simulink model "planner_contral"  (R2023b)
settings: Solver=FixedStepAuto  StartTime=0  StopTime=inf  FixedStep=0.001  RelTol=1e-3
undefined symbols (not defined in the file): aubr, c_factor, cf, cr, iniObsHeading1, iniObsHeading2, iniObsPos1, iniObsPos2, KD_PID_distance, KD_PID_speed, KI_PID_distance, KI_PID_speed, KP_PID_distance, KP_PID_speed, la, lb, LQR_K1, LQR_K2, LQR_K3, LQR_K4, m, rack_displacement, refInfo_obs1, refInfo_obs2, right_wheel_ground, rightWaypoints, tablebr, vubr, vx_break_point
libraries: Solver_SF x1
(part 3 of 8)

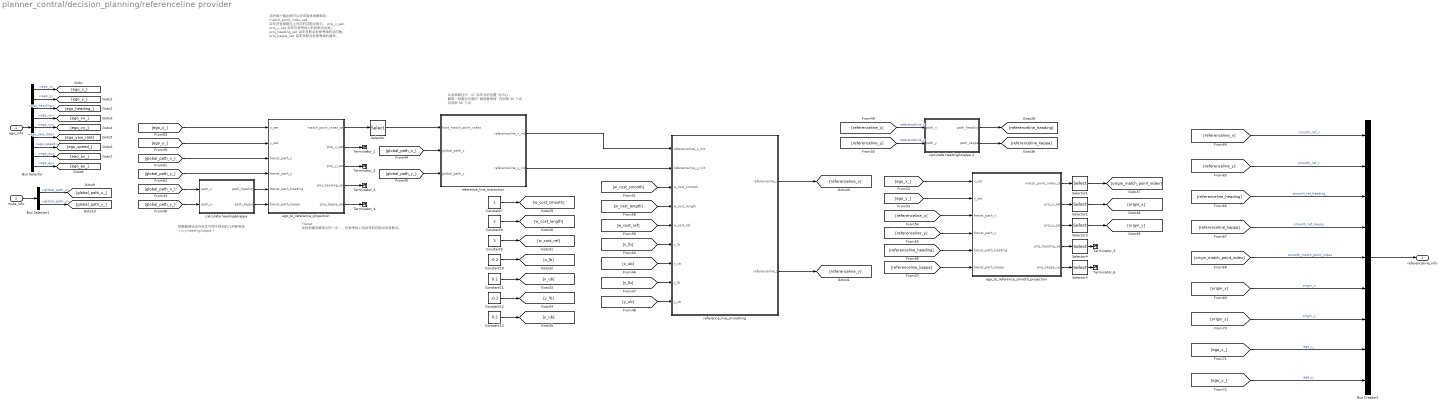
== system planner_contral/decision_planning/referenceline provider ==
  note: 从全局路径中，以“自车当前位置”为中心，
      | 截取一段固定长度的“局部参考线”
      | 向后取 30 个点
      | 向前取 90 个点
  note: 这时每个输出都可以非常具体地解释成：
      | match_point_index_set
      | 自车在全局路径上对应的匹配点索引。
      | proj_x_set, proj_y_set
      | 自车在参考线上的投影点坐标。
      | proj_heading_set
      | 自车投影点处参考线的切向角。
      | proj_kappa_set
      | 自车投影点处参考线的曲率。
  note: Frenet 坐标构建前最核心的一步：在参考线上找自车的匹配点和投影点。
  note: 把离散路径点升级生可用于规划的几何参考线
      | （x,y,heading,kappa）
  ego_info : Inport
  route_info : Inport  Port=2
  Bus Creator2 : BusCreator  Inputs=9
  Bus Selector : BusSelector  OutputSignals=ego_x,ego_y,ego_heading,ego_vx,ego_vy,ego_yaw_rate,ego_speed,ego_ax,ego_ay
  Bus Selector1 : BusSelector  OutputSignals=global_path_x,global_path_y
  Constant10 : Constant  Value=-0.2
  Constant11 : Constant  Value=0.2
  Constant12 : Constant  Value=-0.2
  Constant13 : Constant  Value=0.2
  Constant7 : Constant
  Constant8 : Constant  Value=2
  Constant9 : Constant  Value=3
  Selector{,1..5} (6 alike) : Selector  InputPortWidth=128  IndexOptions=Index vector (dialog)  Indices=1  OutputSizes=1
  Terminator_{1..6} (6 alike) : Terminator
  calculate heading&kappa : MATLAB Function  TreatAsAtomicUnit=on
  calculate heading&kappa 2 : MATLAB Function  TreatAsAtomicUnit=on
  ego_to_reference_projection : MATLAB Function  TreatAsAtomicUnit=on
  ego_to_reference_smooth_projection : MATLAB Function  TreatAsAtomicUnit=on
  reference_line_extraction : MATLAB Function  TreatAsAtomicUnit=on
  reference_line_smoothing : MATLAB Function  TreatAsAtomicUnit=on
  referenceline_info : Outport
  wires:
  ego_info/1 -> Bus Selector/1
  Bus Selector/7 -> [ego_speed_]  "<ego_speed>"
  Bus Selector/8 -> [eao_ax_]  "<ego_ax>"
  Bus Selector/9 -> [ego_ay_]  "<ego_ay>"
  Bus Selector/1 -> [ego_x_]  "<ego_x>"
  Bus Selector/2 -> [ego_y_]  "<ego_y>"
  Bus Selector/3 -> [ego_heading_]  "<ego_heading>"
  Bus Selector/4 -> [ego_vx_]  "<ego_vx>"
  Bus Selector/5 -> [ego_vy_]  "<ego_vy>"
  Bus Selector/6 -> [ego_yaw_rate]  "<ego_yaw_rate>"
  route_info/1 -> Bus Selector1/1
  Bus Selector1/1 -> [global_path_x_]  "<global_path_x>"
  Bus Selector1/2 -> [global_path_y_]  "<global_path_y>"
  Constant8/1 -> [w_cost_length]
  Constant11/1 -> [x_ub]
  [w_cost_ref] -> reference_line_smoothing/5(w_cost_ref)
  [y_lb] -> reference_line_smoothing/8(y_lb)
  [w_cost_smooth] -> reference_line_smoothing/3(w_cost_smooth)
  Constant9/1 -> [w_cost_ref]
  Constant10/1 -> [x_lb]
  reference_line_smoothing/2(referenceline_y) -> [referenceline_y]
  [global_path_y_] -> reference_line_extraction/3(global_path_y)
  [ego_x_] -> ego_to_reference_smooth_projection/1(x_set)
  calculate heading&kappa/1(path_heading) -> ego_to_reference_projection/5(frenet_path_heading)
  [ego_x_] -> ego_to_reference_projection/1(x_set)
  Constant7/1 -> [w_cost_smooth]
  Constant13/1 -> [y_ub]
  ego_to_reference_smooth_projection/5(proj_kappa_set) -> Selector5/1
  [referenceline_kappa] -> ego_to_reference_smooth_projection/6(frenet_path_kappa)
  ego_to_reference_projection/3(proj_y_set) -> Terminator_2/1
  [referenceline_y] -> ego_to_reference_smooth_projection/4(frenet_path_y)
  [referenceline_y] -> calculate heading&kappa 2/2(path_y)  "referenceline_y"
  [global_path_x_] -> ego_to_reference_projection/3(frenet_path_x)
  [global_path_y_] -> ego_to_reference_projection/4(frenet_path_y)
  [x_ub] -> reference_line_smoothing/7(x_ub)
  [global_path_x_] -> calculate heading&kappa/1(path_x)
  reference_line_extraction/2(referenceline_y_init) -> reference_line_smoothing/2(referenceline_y_init)
  ego_to_reference_projection/5(proj_kappa_set) -> Terminator_4/1
  ego_to_reference_projection/4(proj_heading_set) -> Terminator_3/1
  calculate heading&kappa 2/1(path_heading) -> [referenceline_heading]
  ego_to_reference_projection/2(proj_x_set) -> Terminator_1/1
  reference_line_smoothing/1(referenceline_x) -> [referenceline_x]
  Selector3/1 -> [origin_y]
  Selector2/1 -> [origin_x]
  ego_to_reference_smooth_projection/4(proj_heading_set) -> Selector4/1
  calculate heading&kappa 2/2(path_kappa) -> [referenceline_kappa]
  [referenceline_x] -> calculate heading&kappa 2/1(path_x)  "referenceline_x"
  [ego_y_] -> ego_to_reference_projection/2(y_set)
  [x_lb] -> reference_line_smoothing/6(x_lb)
  [referenceline_heading] -> ego_to_reference_smooth_projection/5(frenet_path_heading)
  ego_to_reference_smooth_projection/2(proj_x_set) -> Selector2/1
  calculate heading&kappa/2(path_kappa) -> ego_to_reference_projection/6(frenet_path_kappa)
  [y_ub] -> reference_line_smoothing/9(y_ub)
  [referenceline_x] -> ego_to_reference_smooth_projection/3(frenet_path_x)
  ego_to_reference_smooth_projection/1(match_point_index_set) -> Selector1/1
  [global_path_x_] -> reference_line_extraction/2(global_path_x)
  Selector5/1 -> Terminator_6/1
  reference_line_extraction/1(referenceline_x_init) -> reference_line_smoothing/1(referenceline_x_init)
  Selector4/1 -> Terminator_5/1
  [global_path_y_] -> calculate heading&kappa/2(path_y)
  ego_to_reference_smooth_projection/3(proj_y_set) -> Selector3/1
  ego_to_reference_projection/1(match_point_index_set) -> Selector/1
  Selector/1 -> reference_line_extraction/1(host_match_point_index)
  Constant12/1 -> [y_lb]
  [w_cost_length] -> reference_line_smoothing/4(w_cost_length)
  [ego_y_] -> ego_to_reference_smooth_projection/2(y_set)
  Selector1/1 -> [origin_match_point_index]
  [origin_match_point_index] -> Bus Creator2/5  "smooth_match_point_index"
  [ego_y_] -> Bus Creator2/9  "ego_y_"
  [ego_x_] -> Bus Creator2/8  "ego_x_"
  [referenceline_x] -> Bus Creator2/1  "smooth_ref_x"
  [referenceline_heading] -> Bus Creator2/3  "smooth_ref_heading_"
  [origin_x] -> Bus Creator2/6  "origin_x"
  [referenceline_kappa] -> Bus Creator2/4  "smooth_ref_kappa_"
  [origin_y] -> Bus Creator2/7  "origin_y"
  [referenceline_y] -> Bus Creator2/2  "smooth_ref_y"
  Bus Creator2/1 -> referenceline_info/1

== system planner_contral/control module/control main/chassic steering system ==
  LQR_final_angle : Inport
  Constant : Constant  Value=la
  Constant1 : Constant  Value=lb
  Constant17 : Constant  Value=c_factor
  Divide : Product  Inputs=*/
  Gain3 : Gain  Gain=180/pi
  Gain4 : Gain  Gain=360
  MATLAB Function : MATLAB Function  TreatAsAtomicUnit=on
  Saturation : Saturate  UpperLimit=70  LowerLimit=-70
  Saturation1 : Saturate  UpperLimit=1.2217  LowerLimit=-1.2217
  transfer right wheel angle to rack displancement : Lookup_n-D  NumberOfTableDimensions=1  BreakpointsForDimension1=right_wheel_ground  Table=rack_displacement  InternalRulePriority=Speed  RndMeth=Simplest
  lat_steer_sw[deg] : Outport
  wires:
  transfer right wheel angle to rack displancement/1 -> Divide/1
  Constant17/1 -> Divide/2
  Gain4/1 -> lat_steer_sw[deg]/1
  Divide/1 -> Gain4/1
  Saturation/1 -> transfer right wheel angle to rack displancement/1
  Constant/1 -> MATLAB Function/2(la)
  Gain3/1 -> Saturation/1
  Constant1/1 -> MATLAB Function/3(lb)
  LQR_final_angle/1 -> Saturation1/1
  Saturation1/1 -> MATLAB Function/1(u)
  MATLAB Function/1(right_steer) -> Gain3/1

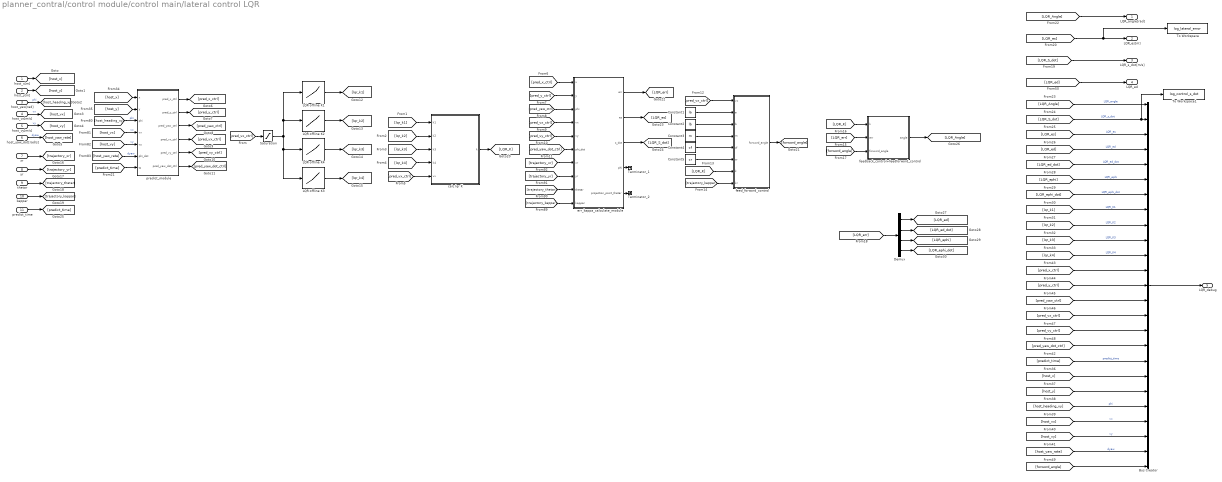
== system planner_contral/control module/control main/lateral control LQR ==
  host_x[m] : Inport
  host_y[m] : Inport  Port=2
  host_yaw[rad] : Inport  Port=3
  host_vx[m/s] : Inport  Port=4
  host_vy[m/s] : Inport  Port=5
  host_yaw_dot[rad/s] : Inport  Port=6
  xr : Inport  Port=7
  yr : Inport  Port=8
  thetar : Inport  Port=9
  kappar : Inport  Port=10
  predict_time : Inport  Port=11
  Bus Creator : BusCreator  Inputs=25
  Constant1 : Constant  Value=la
  Constant2 : Constant  Value=lb
  Constant3 : Constant  Value=m
  Constant4 : Constant  Value=cf
  Constant5 : Constant  Value=cr
  Demux : Demux
  LQR offline K1 : Lookup_n-D  NumberOfTableDimensions=1  BreakpointsForDimension1=vx_break_point  Table=LQR_K1  InternalRulePriority=Speed  RndMeth=Simplest
  LQR offline K2 : Lookup_n-D  NumberOfTableDimensions=1  BreakpointsForDimension1=vx_break_point  Table=LQR_K2  InternalRulePriority=Speed  RndMeth=Simplest
  LQR offline K3 : Lookup_n-D  NumberOfTableDimensions=1  BreakpointsForDimension1=vx_break_point  Table=LQR_K3  InternalRulePriority=Speed  RndMeth=Simplest
  LQR offline K4 : Lookup_n-D  NumberOfTableDimensions=1  BreakpointsForDimension1=vx_break_point  Table=LQR_K4  InternalRulePriority=Speed  RndMeth=Simplest
  Saturation : Saturate  UpperLimit=50  LowerLimit=0
  Terminator_1 : Terminator
  Terminator_2 : Terminator
  To Workspace : ToWorkspace  VariableName=log_lateral_error  SampleTime=-1
  To Workspace1 : ToWorkspace  VariableName=log_control_s_dot  SampleTime=-1
  calc lqr K : MATLAB Function  TreatAsAtomicUnit=on
  err_kappa_calculate_module : MATLAB Function  TreatAsAtomicUnit=on
  feed_forword_control : MATLAB Function  TreatAsAtomicUnit=on
  feedback_control+feedforword_control : MATLAB Function  TreatAsAtomicUnit=on
  predict_module : MATLAB Function  TreatAsAtomicUnit=on
  LQR_angle[rad] : Outport  VectorParamsAs1DForOutWhenUnconnected=off
  LQR_es[m] : Outport  Port=2  VectorParamsAs1DForOutWhenUnconnected=off
  LQR_s_dot[m/s] : Outport  Port=3  VectorParamsAs1DForOutWhenUnconnected=off
  LQR_ed : Outport  Port=4  VectorParamsAs1DForOutWhenUnconnected=off
  LQR_debug : Outport  Port=5  VectorParamsAs1DForOutWhenUnconnected=off
  wires:
  [host_vy] -> predict_module/5(vy)  "vy"
  [host_x] -> predict_module/1(x)
  [host_yaw_rate] -> predict_module/6(phi_dot)  "dyaw"
  [host_vx] -> predict_module/4(vx)  "vx"
  [host_y] -> predict_module/2(y)
  [host_heading_xy] -> predict_module/3(phi)  "phi"
  [predict_time] -> predict_module/7(ts)
  host_x[m]/1 -> [host_x]
  host_y[m]/1 -> [host_y]
  host_yaw[rad]/1 -> [host_heading_xy]  "phi"
  host_vx[m/s]/1 -> [host_vx]  "vx"
  host_vy[m/s]/1 -> [host_vy]  "vy"
  host_yaw_dot[rad/s]/1 -> [host_yaw_rate]  "dyaw"
  predict_module/1(pred_x_ctrl) -> [pred_x_ctrl]
  predict_module/2(pred_y_ctrl) -> [pred_y_ctrl]
  predict_module/3(pred_yaw_ctrl) -> [pred_yaw_ctrl]
  predict_module/4(pred_vx_ctrl) -> [pred_vx_ctrl]
  predict_module/5(pred_vy_ctrl) -> [pred_vy_ctrl]
  predict_module/6(pred_yaw_dot_ctrl) -> [pred_yaw_dot_ctrl]
  [pred_vx_ctrl] -> Saturation/1
  LQR offline K1/1 -> [lqr_k1]
  LQR offline K2/1 -> [lqr_k2]
  LQR offline K4/1 -> [lqr_k3]
  LQR offline K3/1 -> [lqr_k4]
  [pred_vx_ctrl] -> calc lqr K/5(vx)
  [lqr_k4] -> calc lqr K/4(k4)
  [lqr_k3] -> calc lqr K/3(k3)
  [lqr_k2] -> calc lqr K/2(k2)
  [lqr_k1] -> calc lqr K/1(k1)
  [pred_x_ctrl] -> err_kappa_calculate_module/1(x)
  [pred_y_ctrl] -> err_kappa_calculate_module/2(y)
  [pred_yaw_ctrl] -> err_kappa_calculate_module/3("phi ")
  [pred_vx_ctrl] -> err_kappa_calculate_module/4(vx)
  [pred_vy_ctrl] -> err_kappa_calculate_module/5(vy)
  [pred_yaw_dot_ctrl] -> err_kappa_calculate_module/6(phi_dot)
  xr/1 -> [trajectory_xr]
  yr/1 -> [trajectory_yr]
  thetar/1 -> [trajectory_thetar]
  kappar/1 -> [trajectory_kappar]
  [trajectory_xr] -> err_kappa_calculate_module/7(xr)
  [trajectory_yr] -> err_kappa_calculate_module/8(yr)
  [trajectory_kappar] -> err_kappa_calculate_module/10(kappar)
  [trajectory_thetar] -> err_kappa_calculate_module/9(thetar)
  [pred_vx_ctrl] -> feed_forword_control/1(vx)
  Constant1/1 -> feed_forword_control/2(a)
  Constant2/1 -> feed_forword_control/3(b)
  Constant3/1 -> feed_forword_control/4(m)
  Constant4/1 -> feed_forword_control/5(cf)
  Constant5/1 -> feed_forword_control/6(cr)
  calc lqr K/1(k) -> [LQR_K]
  [LQR_K] -> feed_forword_control/7(k)
  [trajectory_kappar] -> feed_forword_control/8(kr)
  feed_forword_control/1(forword_angle) -> [forword_angle]
  err_kappa_calculate_module/1(err) -> [LQR_err]
  [LQR_err] -> feedback_control+feedforword_control/2(err)
  [LQR_K] -> feedback_control+feedforword_control/1(k)
  [forword_angle] -> feedback_control+feedforword_control/3(forword_angle)
  [LQR_err] -> Demux/1
  err_kappa_calculate_module/2(es) -> [LQR_es]
  err_kappa_calculate_module/3(s_dot) -> [LQR_S_dot]
  [LQR_S_dot] -> LQR_s_dot[m/s]/1
  Saturation/1 -> LQR offline K3/1, LQR offline K4/1, LQR offline K2/1, LQR offline K1/1
  predict_time/1 -> [predict_time]
  Bus Creator/1 -> LQR_debug/1
  feedback_control+feedforword_control/1(angle) -> [LQR_Angle]
  [LQR_Angle] -> LQR_angle[rad]/1
  [LQR_Angle] -> Bus Creator/1  "LQR_angle"
  [LQR_S_dot] -> To Workspace1/1, Bus Creator/2  "LQR_s_dot"
  [LQR_es] -> Bus Creator/3  "LQR_es"
  Demux/1 -> [LQR_ed]
  Demux/2 -> [LQR_ed_dot]
  Demux/3 -> [LQR_ephi]
  Demux/4 -> [LQR_ephi_dot]
  [LQR_ed] -> Bus Creator/4  "LQR_ed"
  [LQR_ed_dot] -> Bus Creator/5  "LQR_ed_dot"
  [LQR_ephi] -> Bus Creator/6  "LQR_ephi"
  [LQR_ephi_dot] -> Bus Creator/7  "LQR_ephi_dot"
  [lqr_k1] -> Bus Creator/8  "LQR_K1"
  [lqr_k2] -> Bus Creator/9  "LQR_K2"
  [lqr_k3] -> Bus Creator/10  "LQR_K3"
  [lqr_k4] -> Bus Creator/11  "LQR_K4"
  [pred_x_ctrl] -> Bus Creator/12
  [pred_y_ctrl] -> Bus Creator/13
  [pred_yaw_ctrl] -> Bus Creator/14
  [pred_vx_ctrl] -> Bus Creator/15
  [pred_vy_ctrl] -> Bus Creator/16
  [pred_yaw_dot_ctrl] -> Bus Creator/17
  [predict_time] -> Bus Creator/18  "predict_time"
  [host_x] -> Bus Creator/19
  [host_y] -> Bus Creator/20
  [host_heading_xy] -> Bus Creator/21  "phi"
  [host_vx] -> Bus Creator/22  "vx"
  [host_vy] -> Bus Creator/23  "vy"
  [host_yaw_rate] -> Bus Creator/24  "dyaw"
  [forword_angle] -> Bus Creator/25
  [LQR_ed] -> LQR_ed/1
  err_kappa_calculate_module/4(phi) -> Terminator_1/1
  err_kappa_calculate_module/5(projection_point_thetar) -> Terminator_2/1
  [LQR_es] -> To Workspace/1, LQR_es[m]/1

== system planner_contral/control module/control main/longitudinal control double PID ==
  s_err[m] : Inport
  speed_desire[m/s] : Inport  Port=2
  accelerate desire[m/s^2] : Inport  Port=3
  host_speed[m/s] : Inport  Port=4
  host_s_dot[m/s] : Inport  Port=5
  KP_PID_distance : Inport  Port=6
  KI_PID_distance : Inport  Port=7
  KD_PID_distance : Inport  Port=8
  KP_PID_speed : Inport  Port=9
  KI_PID_speed : Inport  Port=10
  KD_PID_speed : Inport  Port=11
  2-D Lookup Table : Lookup_n-D  BreakpointsForDimension1=vubr  BreakpointsForDimension2=aubr  Table=tablebr  InternalRulePriority=Speed  RndMeth=Simplest
      settings: InputPortMap=u0,u1
  Add : Sum  Inputs=++-
  Add1 : Sum
  Bus Creator : BusCreator  Inputs=9
  Discrete Filter : DiscreteFilter
  MATLAB Function1 : MATLAB Function  TreatAsAtomicUnit=on
  Saturation : Saturate  UpperLimit=45  LowerLimit=-45
  Saturation1 : Saturate  UpperLimit=5  LowerLimit=-8
  To Workspace1 : ToWorkspace  VariableName=log_s_error  SampleTime=-1
  To Workspace3 : ToWorkspace  VariableName=log_host_s_dot  SaveFormat=Timeseries  SampleTime=-1
  To Workspace4 : ToWorkspace  VariableName=log_speed_desire  SampleTime=-1
  To Workspace5 : ToWorkspace  VariableName=log_accel_desire  SampleTime=-1
  discrete pid : Subsystem
  discrete pid1 : Subsystem
  throttle : Outport
  brake : Outport  Port=2
  longitudinal_debug : Outport  Port=3
  wires:
  2-D Lookup Table/1 -> MATLAB Function1/1(u)
  s_err[m]/1 -> To Workspace1/1, [s_err]
  speed_desire[m/s]/1 -> To Workspace4/1, [speed_desire]
  accelerate desire[m/s^2]/1 -> To Workspace5/1, [accelerate_desire]
  KP_PID_distance/1 -> [KP_PID_distance]
  KI_PID_distance/1 -> [KI_PID_distance]
  KD_PID_distance/1 -> [KD_PID_distance]
  KP_PID_speed/1 -> [KP_PID_speed]
  KI_PID_speed/1 -> [KI_PID_speed]
  KD_PID_speed/1 -> [KD_PID_speed]
  [s_err] -> Discrete Filter/1
  host_speed[m/s]/1 -> [host_speed]
  [speed_desire] -> Add/2
  Add/1 -> Saturation/1
  Saturation/1 -> discrete pid1/1(err)
  discrete pid1/1(pid_out) -> Add1/1
  [accelerate_desire] -> Add1/2
  Add1/1 -> Saturation1/1
  Saturation1/1 -> 2-D Lookup Table/2
  host_s_dot[m/s]/1 -> [host_s_dot]
  [host_s_dot] -> To Workspace3/1, Add/3
  [host_speed] -> 2-D Lookup Table/1
  MATLAB Function1/1(throttle) -> throttle/1
  MATLAB Function1/2(brake) -> brake/1
  [KP_PID_distance] -> Bus Creator/1  "KP_PID_distance"
  [KI_PID_distance] -> Bus Creator/2  "KI_PID_distance"
  [KD_PID_distance] -> Bus Creator/3  "KD_PID_distance"
  [KP_PID_speed] -> Bus Creator/4  "KP_PID_speed"
  [KI_PID_speed] -> Bus Creator/5  "KI_PID_speed"
  [KD_PID_speed] -> Bus Creator/6  "KD_PID_speed"
  [host_speed] -> Bus Creator/7  "host_speed"
  [s_err] -> Bus Creator/8  "s_err"
  [host_s_dot] -> Bus Creator/9  "host_s_dot"
  Bus Creator/1 -> longitudinal_debug/1
  Discrete Filter/1 -> discrete pid/1(err)
  [KP_PID_distance] -> discrete pid/2(kp)
  [KI_PID_distance] -> discrete pid/3(ki)
  [KD_PID_distance] -> discrete pid/4(kd)
  [KP_PID_speed] -> discrete pid1/2(kp)
  [KI_PID_speed] -> discrete pid1/3(ki)
  [KD_PID_speed] -> discrete pid1/4(kd)
  discrete pid/1(pid_out) -> Add/1

== system planner_contral/control module/control main/understeer compensate ==
  LQR_angle : Inport
  lateral err : Inport  Port=2
  Add : Sum  Inputs=+-
  Gain : Gain  Gain=0.01
  Manual Switch : ManualSwitch
  LQR_final_angle : Outport
  wires:
  lateral err/1 -> Gain/1
  Add/1 -> Manual Switch/2
  Manual Switch/1 -> LQR_final_angle/1
  LQR_angle/1 -> Add/1, Manual Switch/1
  Gain/1 -> Add/2

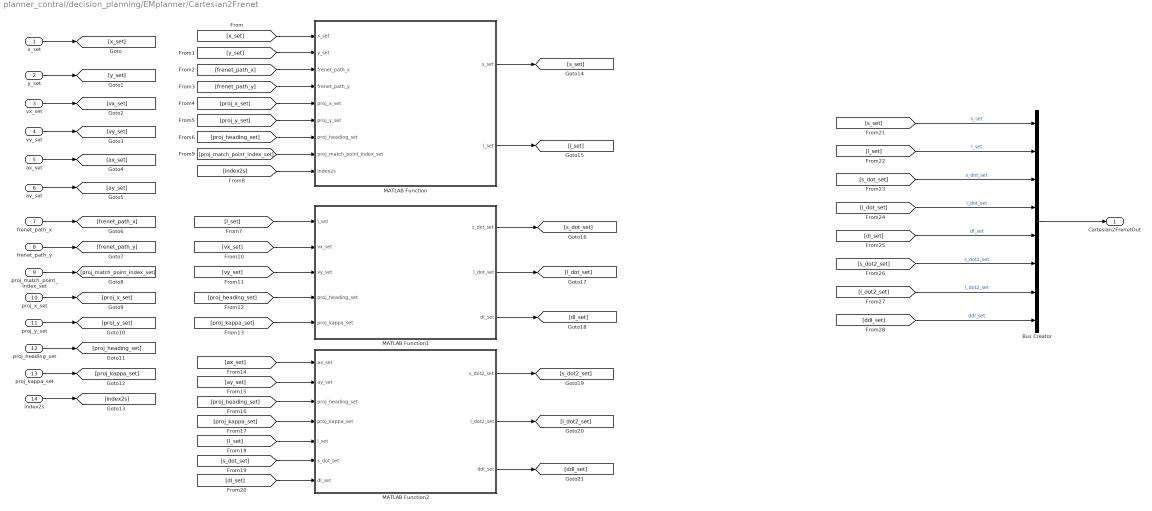
== system planner_contral/decision_planning/EMplanner/Cartesian2Frenet ==
  x_set : Inport
  y_set : Inport  Port=2
  vx_set : Inport  Port=3
  vy_set : Inport  Port=4
  ax_set : Inport  Port=5
  ay_set : Inport  Port=6
  frenet_path_x : Inport  Port=7
  frenet_path_y : Inport  Port=8
  proj_match_point_index_set : Inport  Port=9
  proj_x_set : Inport  Port=10
  proj_y_set : Inport  Port=11
  proj_heading_set : Inport  Port=12
  proj_kappa_set : Inport  Port=13
  index2s : Inport  Port=14
  Bus Creator : BusCreator  Inputs=8
  MATLAB Function : MATLAB Function  TreatAsAtomicUnit=on
  MATLAB Function1 : MATLAB Function  TreatAsAtomicUnit=on
  MATLAB Function2 : MATLAB Function  TreatAsAtomicUnit=on
  Cartesian2FrenetOut : Outport
  wires:
  x_set/1 -> [x_set]
  y_set/1 -> [y_set]
  vx_set/1 -> [vx_set]
  vy_set/1 -> [vy_set]
  ax_set/1 -> [ax_set]
  ay_set/1 -> [ay_set]
  frenet_path_x/1 -> [frenet_path_x]
  frenet_path_y/1 -> [frenet_path_y]
  proj_match_point_index_set/1 -> [proj_match_point_index_set]
  proj_x_set/1 -> [proj_x_set]
  proj_y_set/1 -> [proj_y_set]
  proj_heading_set/1 -> [proj_heading_set]
  proj_kappa_set/1 -> [proj_kappa_set]
  index2s/1 -> [index2s]
  [x_set] -> MATLAB Function/1(x_set)
  [y_set] -> MATLAB Function/2(y_set)
  [frenet_path_x] -> MATLAB Function/3(frenet_path_x)
  [frenet_path_y] -> MATLAB Function/4(frenet_path_y)
  [proj_x_set] -> MATLAB Function/5(proj_x_set)
  [proj_match_point_index_set] -> MATLAB Function/8(proj_match_point_index_set)
  [proj_y_set] -> MATLAB Function/6(proj_y_set)
  [proj_heading_set] -> MATLAB Function/7(proj_heading_set)
  [index2s] -> MATLAB Function/9(index2s)
  MATLAB Function/1(s_set) -> [s_set]
  MATLAB Function/2(l_set) -> [l_set]
  [l_set] -> MATLAB Function1/1(l_set)
  [vx_set] -> MATLAB Function1/2(vx_set)
  [vy_set] -> MATLAB Function1/3(vy_set)
  [proj_heading_set] -> MATLAB Function1/4(proj_heading_set)
  [proj_kappa_set] -> MATLAB Function1/5(proj_kappa_set)
  [ax_set] -> MATLAB Function2/1(ax_set)
  [ay_set] -> MATLAB Function2/2(ay_set)
  [proj_heading_set] -> MATLAB Function2/3(proj_heading_set)
  [proj_kappa_set] -> MATLAB Function2/4(proj_kappa_set)
  [l_set] -> MATLAB Function2/5(l_set)
  MATLAB Function1/1(s_dot_set) -> [s_dot_set]
  MATLAB Function1/2(l_dot_set) -> [l_dot_set]
  MATLAB Function1/3(dl_set) -> [dl_set]
  [s_dot_set] -> MATLAB Function2/6(s_dot_set)
  [dl_set] -> MATLAB Function2/7(dl_set)
  MATLAB Function2/1(s_dot2_set) -> [s_dot2_set]
  MATLAB Function2/2(l_dot2_set) -> [l_dot2_set]
  MATLAB Function2/3(ddl_set) -> [ddl_set]
  [s_set] -> Bus Creator/1  "s_set"
  [l_set] -> Bus Creator/2  "l_set"
  [s_dot_set] -> Bus Creator/3  "s_dot_set"
  [l_dot_set] -> Bus Creator/4  "l_dot_set"
  [dl_set] -> Bus Creator/5  "dl_set"
  [s_dot2_set] -> Bus Creator/6  "s_dot2_set"
  [l_dot2_set] -> Bus Creator/7  "l_dot2_set"
  [ddl_set] -> Bus Creator/8  "ddl_set"
  Bus Creator/1 -> Cartesian2FrenetOut/1

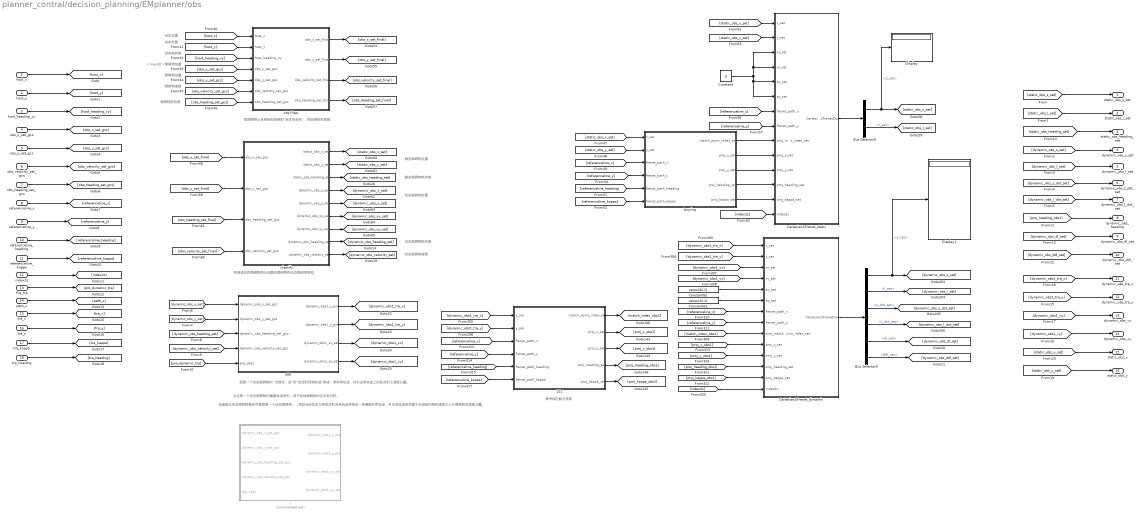
== system planner_contral/decision_planning/EMplanner/obs ==
  note: 参考线匹配与投影
  note: 该函数从动态障碍物集合中提取第一个动态障碍物，将其当前状态与预给定的未来轨迹拼接成一条离散时序轨迹，并为该轨迹附加基于当前航向角和速度大小计算得到的速度分量。
  note: 生成第一个动态障碍物的离散轨迹序列，用于后续障碍物时空关系分析。
  note: 把第一个动态障碍物的“当前状态”和“给定的预测轨迹”拼成一条时序轨迹，并为这条轨迹上的各点附上速度分量。
  note: 静态障碍物位置
  note: 把筛选后的障碍物再分成静态障碍物和动态障碍物两类。
  note: 把障碍物从全局坐标转换到“自车坐标系”，然后做矩形裁剪
  note: 自车位置
  note: 自车位置
  note: 自车航向角
  note: （max32）障碍物位置
  note: 障碍物位置
  note: 障碍物速度
  note: 障碍物航向角
  note: 静态障碍物航向角
  note: 动态障碍物位置
  note: 动态障碍物航向角
  note: 动态障碍物速度
  host_x : Inport
  host_y : Inport  Port=2
  host_heading_xy : Inport  Port=3
  obs_x_set_gcs : Inport  Port=4
  obs_y_set_gcs : Inport  Port=5
  obs_velocity_set_gcs : Inport  Port=6
  obs_heading_set_gcs : Inport  Port=7
  referenceline_x : Inport  Port=8
  referenceline_y : Inport  Port=9
  referenceline_heading : Inport  Port=10
  referenceline_kappa : Inport  Port=11
  index2s : Inport  Port=12
  Pre_tra : Inport  Port=13
  path_s : Inport  Port=14
  tra_x : Inport  Port=15
  tra_y : Inport  Port=16
  tra_kappa : Inport  Port=17
  tra_heaidng : Inport  Port=18
  000 : MATLAB Function  TreatAsAtomicUnit=on
  1 : MATLAB Function  Commented=on  TreatAsAtomicUnit=on
  111 : MATLAB Function  TreatAsAtomicUnit=on
  Bus Selector5 : BusSelector  OutputSignals=s_set,l_set
  Bus Selector9 : BusSelector  OutputSignals=s_set,l_set,s_dot_set,l_dot_set,dl_set,ddl_set
  Cartesian2Frenet_dynamic : Subsystem
  Cartesian2Frenet_static : Subsystem
  Constant : Constant  Value=0
  Constant62 : Constant  Value=zeros(32,1)
  Constant63 : Constant  Value=zeros(32,1)
  Display : Display
  Display1 : Display
  classify : MATLAB Function  TreatAsAtomicUnit=on
  obs filter : MATLAB Function  TreatAsAtomicUnit=on
  touying : MATLAB Function  TreatAsAtomicUnit=on
  static_obs_s_set : Outport
  static_obs_l_set : Outport  Port=2
  static_obs_heading_set : Outport  Port=3
  dynamic_obs_s_set : Outport  Port=4
  dynamic_obs_l_set : Outport  Port=5
  dynamic_obs_s_dot_set : Outport  Port=6
  dynamic_obs_l_dot_set : Outport  Port=7
  dynamic_obs_heading : Outport  Port=8
  dynamic_obs_dl_set : Outport  Port=9
  dynamic_obs_ddl_set : Outport  Port=10
  dynamic_obs_tra_x : Outport  Port=11
  dynamic_obs_tra_y : Outport  Port=12
  dynamic_obs_vx : Outport  Port=13
  dynamic_obs_vy : Outport  Port=14
  static_obs_x : Outport  Port=15
  static_obs_y : Outport  Port=16
  wires:
  Constant/1 -> Cartesian2Frenet_static/6(ay_set), Cartesian2Frenet_static/5(ax_set), Cartesian2Frenet_static/4(vy_set), Cartesian2Frenet_static/3(vx_set)
  [obs_x_set_gcs] -> obs filter/4(obs_x_set_gcs)
  [index2s] -> Cartesian2Frenet_static/14(index2s)
  [referenceline_y] -> Cartesian2Frenet_static/8(frenet_path_y)
  touying/5(proj_kappa_set) -> Cartesian2Frenet_static/13(proj_kappa_set)
  touying/4(proj_heading_set) -> Cartesian2Frenet_static/12(proj_heading_set)
  [referenceline_x] -> touying/3(frenet_path_x)
  obs filter/1(obs_x_set_final) -> [obs_x_set_final]
  obs filter/4(obs_heading_set_final) -> [obs_heading_set_final]
  [host_heading_xy] -> obs filter/3(host_heading_xy)
  classify/6(dynamic_obs_vx_set) -> [dynamic_obs_vx_set]
  [obs_y_set_final] -> classify/2(obs_y_set_gcs)
  classify/7(dynamic_obs_vy_set) -> [dynamic_obs_vy_set]
  [referenceline_y] -> touying/4(frenet_path_y)
  obs filter/3(obs_velocity_set_final) -> [obs_velocity_set_final]
  classify/1(static_obs_x_set) -> [static_obs_x_set]
  [obs_heading_set_gcs] -> obs filter/7(obs_heading_set_gcs)
  [referenceline_kappa] -> touying/6(frenet_path_kappa)
  [static_obs_x_set] -> Cartesian2Frenet_static/1(x_set)
  [static_obs_y_set] -> touying/2(y_set)
  [referenceline_x] -> Cartesian2Frenet_static/7(frenet_path_x)
  [obs_x_set_final] -> classify/1(obs_x_set_gcs)
  [obs_velocity_set_gcs] -> obs filter/6(obs_velocity_set_gcs)
  [host_y] -> obs filter/2(host_y)
  Bus Selector5/2 -> [static_obs_l_set]  "<l_set>"
  [referenceline_heading] -> touying/5(frenet_path_heading)
  obs filter/2(obs_y_set_final) -> [obs_y_set_final]
  Bus Selector5/1 -> Display/1, [static_obs_s_set]  "<s_set>"
  classify/4(dynamic_obs_x_set) -> [dynamic_obs_x_set]
  touying/2(proj_x_set) -> Cartesian2Frenet_static/10(proj_x_set)
  touying/3(proj_y_set) -> Cartesian2Frenet_static/11(proj_y_set)
  classify/5(dynamic_obs_y_set) -> [dynamic_obs_y_set]
  touying/1(match_point_index_set) -> Cartesian2Frenet_static/9(proj_match_point_index_set)
  [host_x] -> obs filter/1(host_x)
  [obs_y_set_gcs] -> obs filter/5(obs_y_set_gcs)
  Cartesian2Frenet_static/1(Cartesian2FrenetOut) -> Bus Selector5/1
  [static_obs_x_set] -> touying/1(x_set)
  classify/2(static_obs_y_set) -> [static_obs_y_set]
  [static_obs_y_set] -> Cartesian2Frenet_static/2(y_set)
  host_x/1 -> [host_x]
  host_y/1 -> [host_y]
  host_heading_xy/1 -> [host_heading_xy]
  obs_x_set_gcs/1 -> [obs_x_set_gcs]
  obs_y_set_gcs/1 -> [obs_y_set_gcs]
  obs_velocity_set_gcs/1 -> [obs_velocity_set_gcs]
  obs_heading_set_gcs/1 -> [obs_heading_set_gcs]
  referenceline_x/1 -> [referenceline_x]
  referenceline_y/1 -> [referenceline_y]
  referenceline_heading/1 -> [referenceline_heading]
  referenceline_kappa/1 -> [referenceline_kappa]
  index2s/1 -> [index2s]
  [static_obs_s_set] -> static_obs_s_set/1
  [static_obs_l_set] -> static_obs_l_set/1
  [dynamic_obs_l_dot_set] -> dynamic_obs_l_dot_set/1
  [dynamic_obs_s_dot_set] -> dynamic_obs_s_dot_set/1
  [dynamic_obs_l_set] -> dynamic_obs_l_set/1
  [dynamic_obs_s_set] -> dynamic_obs_s_set/1
  [obs_velocity_set_final] -> classify/4(obs_velocity_set_gcs)
  [obs_heading_set_final] -> classify/3(obs_heading_set_gcs)
  [index2s] -> Cartesian2Frenet_dynamic/14(index2s)
  000/2(dynamic_obs1_y_pre) -> [dynamic_obs1_tra_y]
  [referenceline_x] -> Cartesian2Frenet_dynamic/7(frenet_path_x)
  [referenceline_kappa] -> 111/6(frenet_path_kappa)
  [proj_y_obs1] -> Cartesian2Frenet_dynamic/11(proj_y_set)
  Bus Selector9/1 -> Display1/1, [dynamic_obs_s_set]  "<s_set>"
  Bus Selector9/3 -> [dynamic_obs_s_dot_set]  "<s_dot_set>"
  [dynamic_obs1_vy] -> Cartesian2Frenet_dynamic/4(vy_set)
  [dynamic_obs1_vx] -> Cartesian2Frenet_dynamic/3(vx_set)
  [proj_heading_obs1] -> Cartesian2Frenet_dynamic/12(proj_heading_set)
  [dynamic_obs1_tra_y] -> 111/2(y_set)
  [referenceline_y] -> 111/4(frenet_path_y)
  [proj_x_obs1] -> Cartesian2Frenet_dynamic/10(proj_x_set)
  Cartesian2Frenet_dynamic/1(Cartesian2FrenetOut) -> Bus Selector9/1
  Bus Selector9/4 -> [dynamic_obs_l_dot_set]  "<l_dot_set>"
  [match_index_obs1] -> Cartesian2Frenet_dynamic/9(proj_match_point_index_set)
  [dynamic_obs_x_set] -> 000/1(dynamic_obs_x_set_gcs)
  111/3(proj_y_set) -> [proj_y_obs1]
  Constant62/1 -> Cartesian2Frenet_dynamic/5(ax_set)
  000/1(dynamic_obs1_x_pre) -> [dynamic_obs1_tra_x]
  000/3(dynamic_obs1_vx_set) -> [dynamic_obs1_vx]
  111/1(match_point_index_set) -> [match_index_obs1]
  000/4(dynamic_obs1_vy_set) -> [dynamic_obs1_vy]
  Constant63/1 -> Cartesian2Frenet_dynamic/6(ay_set)
  [referenceline_y] -> Cartesian2Frenet_dynamic/8(frenet_path_y)
  [dynamic_obs1_tra_x] -> 111/1(x_set)
  111/5(proj_kappa_set) -> [proj_kappa_obs1]
  Bus Selector9/2 -> [dynamic_obs_l_set]  "<l_set>"
  [dynamic_obs1_tra_y] -> Cartesian2Frenet_dynamic/2(y_set)
  [referenceline_x] -> 111/3(frenet_path_x)
  [proj_kappa_obs1] -> Cartesian2Frenet_dynamic/13(proj_kappa_set)
  [referenceline_heading] -> 111/5(frenet_path_heading)
  111/2(proj_x_set) -> [proj_x_obs1]
  [dynamic_obs1_tra_x] -> Cartesian2Frenet_dynamic/1(x_set)
  111/4(proj_heading_set) -> [proj_heading_obs1]
  Pre_tra/1 -> [pro_dynamic_tra]
  path_s/1 -> [path_s]
  tra_y/1 -> [tra_y]
  tra_x/1 -> [tra_x]
  tra_heaidng/1 -> [tra_heading]
  tra_kappa/1 -> [tra_kappa]
  [dynamic_obs_y_set] -> 000/2(dynamic_obs_y_set_gcs)
  [dynamic_obs_heading_set] -> 000/3(dynamic_obs_heading_set_gcs)
  [dynamic_obs_velocity_set] -> 000/4(dynamic_obs_velocity_set_gcs)
  [pro_dynamic_tra] -> 000/5(pre_obs1)
  classify/8(dynamic_obs_heading_set) -> [dynamic_obs_heading_set]
  classify/9(dynamic_obs_velocity_set) -> [dynamic_obs_velocity_set]
  [proj_heading_obs1] -> dynamic_obs_heading/1
  Bus Selector9/5 -> [dynamic_obs_dl_set]  "<dl_set>"
  Bus Selector9/6 -> [dynamic_obs_ddl_set]  "<ddl_set>"
  [dynamic_obs_dl_set] -> dynamic_obs_dl_set/1
  [dynamic_obs_ddl_set] -> dynamic_obs_ddl_set/1
  classify/3(static_obs_heading_set) -> [static_obs_heading_set]
  [static_obs_heading_set] -> static_obs_heading_set/1
  [dynamic_obs1_vy] -> dynamic_obs_vy/1
  [dynamic_obs1_tra_y] -> dynamic_obs_tra_y/1
  [dynamic_obs1_vx] -> dynamic_obs_vx/1
  [dynamic_obs1_tra_x] -> dynamic_obs_tra_x/1
  [static_obs_x_set] -> static_obs_x/1
  [static_obs_y_set] -> static_obs_y/1

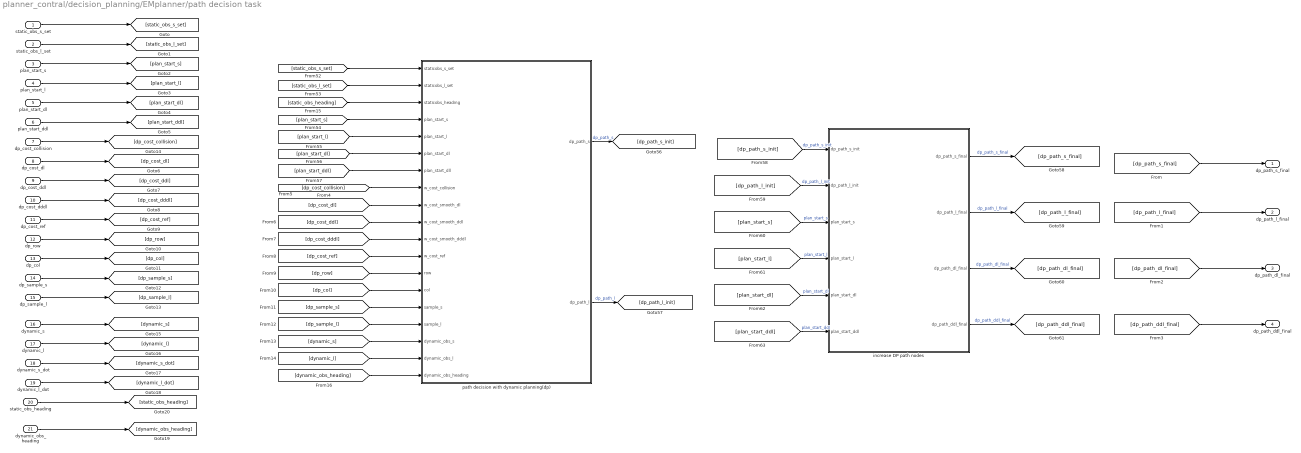
== system planner_contral/decision_planning/EMplanner/path decision task ==
  static_obs_s_set : Inport
  static_obs_l_set : Inport  Port=2
  plan_start_s : Inport  Port=3
  plan_start_l : Inport  Port=4
  plan_start_dl : Inport  Port=5
  plan_start_ddl : Inport  Port=6
  dp_cost_collision : Inport  Port=7
  dp_cost_dl : Inport  Port=8
  dp_cost_ddl : Inport  Port=9
  dp_cost_dddl : Inport  Port=10
  dp_cost_ref : Inport  Port=11
  dp_row : Inport  Port=12
  dp_col : Inport  Port=13
  dp_sample_s : Inport  Port=14
  dp_sample_l : Inport  Port=15
  dynamic_s : Inport  Port=16
  dynamic_l : Inport  Port=17
  dynamic_s_dot : Inport  Port=18
  dynamic_l_dot : Inport  Port=19
  static_obs_heading : Inport  Port=20
  dynamic_obs_heading : Inport  Port=21
  increase DP path nodes : MATLAB Function  TreatAsAtomicUnit=on
  path decision with dynamic planning(dp) : MATLAB Function  TreatAsAtomicUnit=on
  dp_path_s_final : Outport
  dp_path_l_final : Outport  Port=2
  dp_path_dl_final : Outport  Port=3
  dp_path_ddl_final : Outport  Port=4
  wires:
  [plan_start_s] -> path decision with dynamic planning(dp)/4(plan_start_s)
  path decision with dynamic planning(dp)/1(dp_path_s) -> [dp_path_s_init]  "dp_path_s"
  increase DP path nodes/2(dp_path_l_final) -> [dp_path_l_final]  "dp_path_l_final"
  [static_obs_l_set] -> path decision with dynamic planning(dp)/2(staticobs_l_set)
  [plan_start_ddl] -> path decision with dynamic planning(dp)/7(plan_start_dll)
  [plan_start_l] -> path decision with dynamic planning(dp)/5(plan_start_l)
  [static_obs_s_set] -> path decision with dynamic planning(dp)/1(staticobs_s_set)
  [plan_start_dl] -> increase DP path nodes/5(plan_start_dl)  "plan_start_dl"
  increase DP path nodes/4(dp_path_ddl_final) -> [dp_path_ddl_final]  "dp_path_ddl_final"
  increase DP path nodes/1(dp_path_s_final) -> [dp_path_s_final]  "dp_path_s_final"
  increase DP path nodes/3(dp_path_dl_final) -> [dp_path_dl_final]  "dp_path_dl_final"
  path decision with dynamic planning(dp)/2(dp_path_l) -> [dp_path_l_init]  "dp_path_l"
  [plan_start_l] -> increase DP path nodes/4(plan_start_l)  "plan_start_l"
  [plan_start_ddl] -> increase DP path nodes/6(plan_start_ddl)  "plan_start_ddl"
  [plan_start_dl] -> path decision with dynamic planning(dp)/6(plan_start_dl)
  [plan_start_s] -> increase DP path nodes/3(plan_start_s)  "plan_start_s"
  [dp_path_l_init] -> increase DP path nodes/2(dp_path_l_init)  "dp_path_l_init"
  [dp_path_s_init] -> increase DP path nodes/1(dp_path_s_init)  "dp_path_s_init"
  static_obs_s_set/1 -> [static_obs_s_set]
  static_obs_l_set/1 -> [static_obs_l_set]
  plan_start_s/1 -> [plan_start_s]
  plan_start_l/1 -> [plan_start_l]
  plan_start_dl/1 -> [plan_start_dl]
  plan_start_ddl/1 -> [plan_start_ddl]
  [dp_path_s_final] -> dp_path_s_final/1
  [dp_path_l_final] -> dp_path_l_final/1
  [dp_path_dl_final] -> dp_path_dl_final/1
  [dp_path_ddl_final] -> dp_path_ddl_final/1
  [dp_cost_collision] -> path decision with dynamic planning(dp)/8(w_cost_collision)
  [dp_cost_dl] -> path decision with dynamic planning(dp)/9(w_cost_smooth_dl)
  [dp_cost_ddl] -> path decision with dynamic planning(dp)/10(w_cost_smooth_ddl)
  [dp_cost_dddl] -> path decision with dynamic planning(dp)/11(w_cost_smooth_dddl)
  [dp_cost_ref] -> path decision with dynamic planning(dp)/12(w_cost_ref)
  [dp_row] -> path decision with dynamic planning(dp)/13(row)
  [dp_col] -> path decision with dynamic planning(dp)/14(col)
  [dp_sample_s] -> path decision with dynamic planning(dp)/15(sample_s)
  [dp_sample_l] -> path decision with dynamic planning(dp)/16(sample_l)
  dp_cost_dl/1 -> [dp_cost_dl]
  dp_cost_ddl/1 -> [dp_cost_ddl]
  dp_cost_dddl/1 -> [dp_cost_dddl]
  dp_cost_ref/1 -> [dp_cost_ref]
  dp_row/1 -> [dp_row]
  dp_col/1 -> [dp_col]
  dp_sample_l/1 -> [dp_sample_l]
  dp_sample_s/1 -> [dp_sample_s]
  dp_cost_collision/1 -> [dp_cost_collision]
  dynamic_l/1 -> [dynamic_l]
  dynamic_s/1 -> [dynamic_s]
  dynamic_l_dot/1 -> [dynamic_l_dot]
  dynamic_s_dot/1 -> [dynamic_s_dot]
  [dynamic_s] -> path decision with dynamic planning(dp)/17(dynamic_obs_s)
  [dynamic_l] -> path decision with dynamic planning(dp)/18(dynamic_obs_l)
  [static_obs_heading] -> path decision with dynamic planning(dp)/3(staticobs_heading)
  static_obs_heading/1 -> [static_obs_heading]
  dynamic_obs_heading/1 -> [dynamic_obs_heading]
  [dynamic_obs_heading] -> path decision with dynamic planning(dp)/19(dynamic_obs_heading)

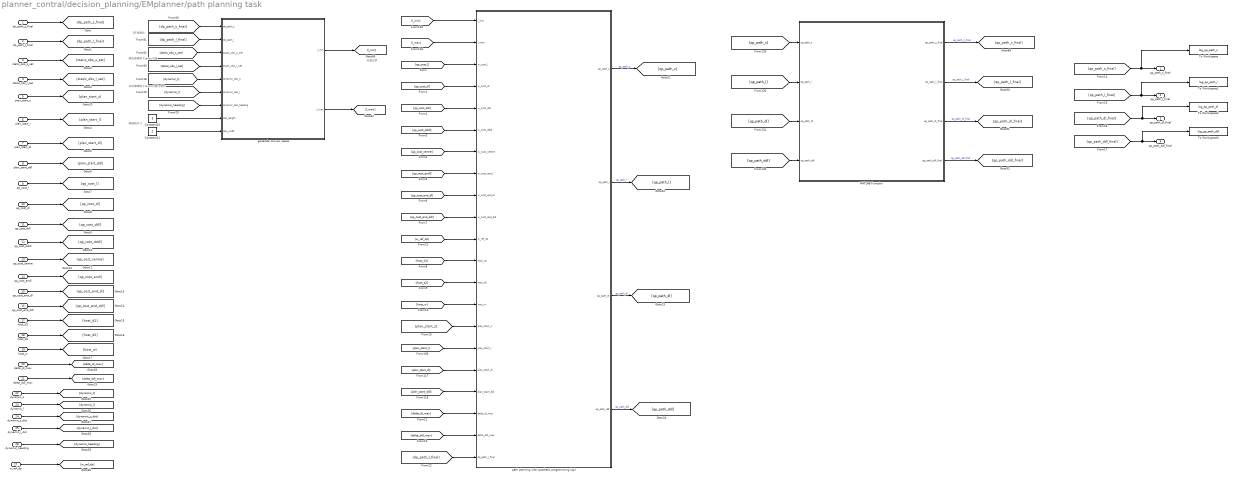
== system planner_contral/decision_planning/EMplanner/path planning task ==
  note: 走廊边界
  note: 障碍物尺寸
  note: 动态障碍物 Frenet 位置与朝向
  note: 静态障碍物 Frenet 位置
  note: DP粗路径
  dp_path_s_final : Inport
  dp_path_l_final : Inport  Port=2
  static_obs_s_set : Inport  Port=3
  static_obs_l_set : Inport  Port=4
  plan_start_s : Inport  Port=5
  plan_start_l : Inport  Port=6
  plan_start_dl : Inport  Port=7
  plan_start_ddl : Inport  Port=8
  qp_cost_l : Inport  Port=9
  qp_cost_dl : Inport  Port=10
  qp_cost_ddl : Inport  Port=11
  qp_cost_dddl : Inport  Port=12
  qp_cost_centre : Inport  Port=13
  qp_cost_endl : Inport  Port=14
  qp_cost_end_dl : Inport  Port=15
  qp_cost_end_ddl : Inport  Port=16
  host_d1 : Inport  Port=17
  host_d2 : Inport  Port=18
  host_w : Inport  Port=19
  delta_dl_max : Inport  Port=20
  delta_ddl_max : Inport  Port=21
  dynamic_s : Inport  Port=22
  dynamic_l : Inport  Port=23
  dynamic_s_dot : Inport  Port=24
  dynamic_l_dot : Inport  Port=25
  dynamic_heading : Inport  Port=26
  w_ref_dp : Inport  Port=27
  Constant10 : Constant  Value=5
  Constant11 : Constant  Value=2
  MATLAB Function : MATLAB Function  TreatAsAtomicUnit=on
  To Workspace : ToWorkspace  VariableName=log_qp_path_s  SampleTime=-1
  To Workspace1 : ToWorkspace  VariableName=log_qp_path_l  SampleTime=-1
  To Workspace2 : ToWorkspace  VariableName=log_qp_path_dl  SampleTime=-1
  To Workspace3 : ToWorkspace  VariableName=log_qp_path_ddl  SampleTime=-1
  generate convex space : MATLAB Function  TreatAsAtomicUnit=on
  path planning with quadratic programming (qp) : MATLAB Function  TreatAsAtomicUnit=on
  qp_path_s_final : Outport
  qp_path_l_final : Outport  Port=2
  qp_path_dl_final : Outport  Port=3
  qp_path_ddl_final : Outport  Port=4
  wires:
  generate convex space/2(l_max) -> [l_max]
  [static_obs_l_set] -> generate convex space/4(static_obs_l_set)
  [dp_path_s_final] -> generate convex space/1(dp_path_s)
  [plan_start_l] -> path planning with quadratic programming (qp)/16(plan_start_l)
  generate convex space/1(l_min) -> [l_min]
  [static_obs_s_set] -> generate convex space/3(static_obs_s_set)
  [dp_path_l_final] -> generate convex space/2(dp_path_l)
  [plan_start_dl] -> path planning with quadratic programming (qp)/17(plan_start_dl)
  [l_max] -> path planning with quadratic programming (qp)/2(l_max)
  [l_min] -> path planning with quadratic programming (qp)/1(l_min)
  [plan_start_ddl] -> path planning with quadratic programming (qp)/18(plan_start_ddl)
  dp_path_s_final/1 -> [dp_path_s_final]
  dp_path_l_final/1 -> [dp_path_l_final]
  static_obs_s_set/1 -> [static_obs_s_set]
  static_obs_l_set/1 -> [static_obs_l_set]
  plan_start_l/1 -> [plan_start_l]
  plan_start_dl/1 -> [plan_start_dl]
  plan_start_ddl/1 -> [plan_start_ddl]
  [qp_cost_l] -> path planning with quadratic programming (qp)/3(w_cost_l)
  [qp_cost_dl] -> path planning with quadratic programming (qp)/4(w_cost_dl)
  [qp_cost_ddl] -> path planning with quadratic programming (qp)/5(w_cost_ddl)
  [qp_cost_dddl] -> path planning with quadratic programming (qp)/6(w_cost_dddl)
  [qp_cost_centre] -> path planning with quadratic programming (qp)/7(w_cost_centre)
  [qp_cost_endl] -> path planning with quadratic programming (qp)/8(w_cost_end_l)
  [qp_cost_end_dl] -> path planning with quadratic programming (qp)/9(w_cost_end_dl)
  [qp_cost_end_ddl] -> path planning with quadratic programming (qp)/10(w_cost_end_ddl)
  [host_d1] -> path planning with quadratic programming (qp)/12(host_d1)
  [host_d2] -> path planning with quadratic programming (qp)/13(host_d2)
  [host_w] -> path planning with quadratic programming (qp)/14(host_w)
  qp_cost_l/1 -> [qp_cost_l]
  qp_cost_dl/1 -> [qp_cost_dl]
  qp_cost_ddl/1 -> [qp_cost_ddl]
  qp_cost_dddl/1 -> [qp_cost_dddl]
  qp_cost_centre/1 -> [qp_cost_centre]
  qp_cost_endl/1 -> [qp_cost_endl]
  qp_cost_end_dl/1 -> [qp_cost_end_dl]
  qp_cost_end_ddl/1 -> [qp_cost_end_ddl]
  host_d1/1 -> [host_d1]
  host_d2/1 -> [host_d2]
  host_w/1 -> [host_w]
  [delta_dl_max] -> path planning with quadratic programming (qp)/19(delta_dl_max)
  [delta_ddl_max] -> path planning with quadratic programming (qp)/20(delta_ddl_max)
  delta_dl_max/1 -> [delta_dl_max]
  delta_ddl_max/1 -> [delta_ddl_max]
  plan_start_s/1 -> [plan_start_s]
  [plan_start_s] -> path planning with quadratic programming (qp)/15(plan_start_s)
  MATLAB Function/1(qp_path_s_final) -> [qp_path_s_final]  "qp_path_s_final"
  MATLAB Function/3(qp_path_dl_final) -> [qp_path_dl_final]  "qp_path_dl_final"
  [qp_path_s] -> MATLAB Function/1(qp_path_s)
  [qp_path_ddl] -> MATLAB Function/4(qp_path_ddl)
  MATLAB Function/2(qp_path_l_final) -> [qp_path_l_final]  "qp_path_l_final"
  [qp_path_dl] -> MATLAB Function/3(qp_path_dl)
  MATLAB Function/4(qp_path_ddl_final) -> [qp_path_ddl_final]  "qp_path_ddl-final"
  [qp_path_l] -> MATLAB Function/2(qp_path_l)
  [qp_path_s_final] -> To Workspace/1, qp_path_s_final/1
  [qp_path_l_final] -> To Workspace1/1, qp_path_l_final/1
  [qp_path_dl_final] -> To Workspace2/1, qp_path_dl_final/1
  [qp_path_ddl_final] -> To Workspace3/1, qp_path_ddl_final/1
  path planning with quadratic programming (qp)/1(qp_path_s) -> [qp_path_s]  "qp_path_s"
  path planning with quadratic programming (qp)/2(qp_path_l) -> [qp_path_l]  "qp_path_l"
  path planning with quadratic programming (qp)/3(qp_path_dl) -> [qp_path_dl]  "qp_path_dl"
  path planning with quadratic programming (qp)/4(qp_path_ddl) -> [qp_path_ddl]  "qp_path_ddl"
  dynamic_l_dot/1 -> [dynamic_l_dot]
  dynamic_l/1 -> [dynamic_l]
  dynamic_s_dot/1 -> [dynamic_s_dot]
  dynamic_s/1 -> [dynamic_s]
  Constant11/1 -> generate convex space/9(obs_width)
  Constant10/1 -> generate convex space/8(obs_length)
  [dynamic_s] -> generate convex space/5(dynamic_obs_s)
  [dynamic_l] -> generate convex space/6(dynamic_obs_l)
  [dynamic_heading] -> generate convex space/7(dynamic_obs_heading)
  dynamic_heading/1 -> [dynamic_heading]
  w_ref_dp/1 -> [w_ref_dp]
  [w_ref_dp] -> path planning with quadratic programming (qp)/11(w_ref_dp)
  [dp_path_l_final] -> path planning with quadratic programming (qp)/21(dp_path_l_final)

== system planner_contral/control module/control main/longitudinal control double PID/discrete pid ==
  err : Inport
  kp : Inport  Port=2
  ki : Inport  Port=3
  kd : Inport  Port=4
  Add2 : Sum  Inputs=+++
  Add3 : Sum
  Add4 : Sum  Inputs=+-
  Delay3 : Delay  DelayLength=1
  Delay4 : Delay  DelayLength=1
  Divide : Product  Inputs=**
  Divide1 : Product  Inputs=**
  Divide2 : Product  Inputs=**
  Gain : Gain  Gain=0.01
  pid_out : Outport
  wires:
  [KD_PID_distance] -> Divide2/2
  err/1 -> Delay4/1, Divide/2, Add3/1, Add4/1
  Divide/1 -> Add2/1
  Divide2/1 -> Add2/3
  Add3/1 -> Gain/1, Divide1/1
  Delay4/1 -> Add4/2
  [KP_PID_distance] -> Divide/1
  Divide1/1 -> Add2/2
  Delay3/1 -> Add3/2
  [KI_PID_distance] -> Divide1/2
  Add4/1 -> Divide2/1
  Add2/1 -> pid_out/1
  kp/1 -> [KP_PID_distance]
  ki/1 -> [KI_PID_distance]
  kd/1 -> [KD_PID_distance]
  Gain/1 -> Delay3/1

== system planner_contral/control module/control main/longitudinal control double PID/discrete pid1 ==
  err : Inport
  kp : Inport  Port=2
  ki : Inport  Port=3
  kd : Inport  Port=4
  Add2 : Sum  Inputs=+++
  Add3 : Sum
  Add4 : Sum  Inputs=+-
  Delay3 : Delay  DelayLength=1
  Delay4 : Delay  DelayLength=1
  Divide : Product  Inputs=**
  Divide1 : Product  Inputs=**
  Divide2 : Product  Inputs=**
  Gain : Gain  Gain=0.01
  pid_out : Outport
  wires:
  Gain/1 -> Delay3/1
  kd/1 -> [KD_PID_distance]
  ki/1 -> [KI_PID_distance]
  kp/1 -> [KP_PID_distance]
  Add2/1 -> pid_out/1
  Add4/1 -> Divide2/1
  [KI_PID_distance] -> Divide1/2
  Delay3/1 -> Add3/2
  Divide1/1 -> Add2/2
  [KP_PID_distance] -> Divide/1
  Delay4/1 -> Add4/2
  Add3/1 -> Divide1/1, Gain/1
  Divide2/1 -> Add2/3
  Divide/1 -> Add2/1
  err/1 -> Add4/1, Add3/1, Divide/2, Delay4/1
  [KD_PID_distance] -> Divide2/2

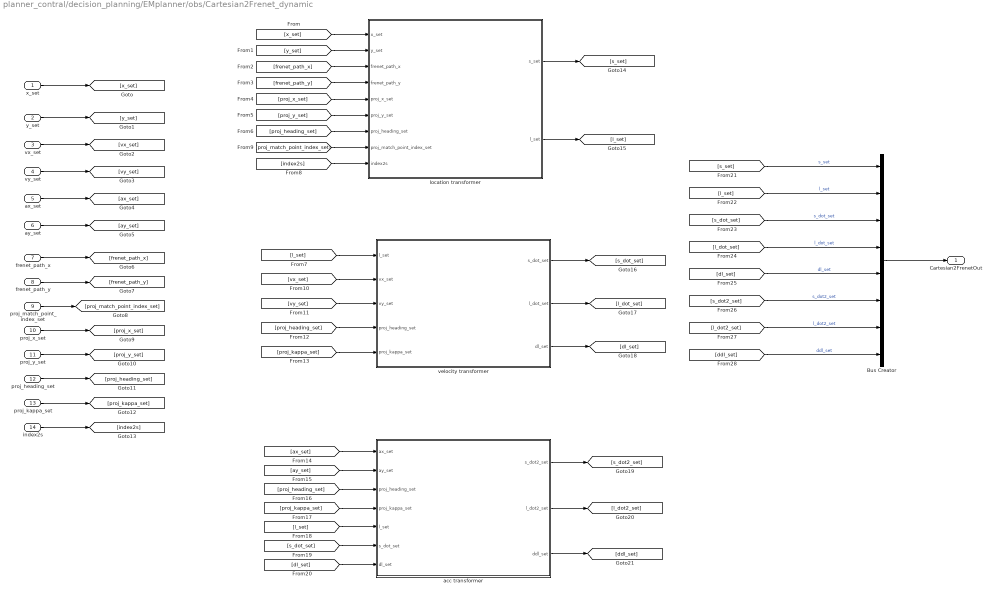
== system planner_contral/decision_planning/EMplanner/obs/Cartesian2Frenet_dynamic ==
  x_set : Inport
  y_set : Inport  Port=2
  vx_set : Inport  Port=3
  vy_set : Inport  Port=4
  ax_set : Inport  Port=5
  ay_set : Inport  Port=6
  frenet_path_x : Inport  Port=7
  frenet_path_y : Inport  Port=8
  proj_match_point_index_set : Inport  Port=9
  proj_x_set : Inport  Port=10
  proj_y_set : Inport  Port=11
  proj_heading_set : Inport  Port=12
  proj_kappa_set : Inport  Port=13
  index2s : Inport  Port=14
  Bus Creator : BusCreator  Inputs=8
  acc transformer : MATLAB Function  TreatAsAtomicUnit=on
  location transformer : MATLAB Function  TreatAsAtomicUnit=on
  velocity transformer : MATLAB Function  TreatAsAtomicUnit=on
  Cartesian2FrenetOut : Outport
  wires:
  Bus Creator/1 -> Cartesian2FrenetOut/1
  [ddl_set] -> Bus Creator/8  "ddl_set"
  [l_dot2_set] -> Bus Creator/7  "l_dot2_set"
  [s_dot2_set] -> Bus Creator/6  "s_dot2_set"
  [dl_set] -> Bus Creator/5  "dl_set"
  [l_dot_set] -> Bus Creator/4  "l_dot_set"
  [s_dot_set] -> Bus Creator/3  "s_dot_set"
  [l_set] -> Bus Creator/2  "l_set"
  [s_set] -> Bus Creator/1  "s_set"
  acc transformer/3(ddl_set) -> [ddl_set]
  acc transformer/2(l_dot2_set) -> [l_dot2_set]
  acc transformer/1(s_dot2_set) -> [s_dot2_set]
  [dl_set] -> acc transformer/7(dl_set)
  [s_dot_set] -> acc transformer/6(s_dot_set)
  velocity transformer/3(dl_set) -> [dl_set]
  velocity transformer/2(l_dot_set) -> [l_dot_set]
  velocity transformer/1(s_dot_set) -> [s_dot_set]
  [l_set] -> acc transformer/5(l_set)
  [proj_kappa_set] -> acc transformer/4(proj_kappa_set)
  [proj_heading_set] -> acc transformer/3(proj_heading_set)
  [ay_set] -> acc transformer/2(ay_set)
  [ax_set] -> acc transformer/1(ax_set)
  [proj_kappa_set] -> velocity transformer/5(proj_kappa_set)
  [proj_heading_set] -> velocity transformer/4(proj_heading_set)
  [vy_set] -> velocity transformer/3(vy_set)
  [vx_set] -> velocity transformer/2(vx_set)
  [l_set] -> velocity transformer/1(l_set)
  location transformer/2(l_set) -> [l_set]
  location transformer/1(s_set) -> [s_set]
  [index2s] -> location transformer/9(index2s)
  [proj_heading_set] -> location transformer/7(proj_heading_set)
  [proj_y_set] -> location transformer/6(proj_y_set)
  [proj_match_point_index_set] -> location transformer/8(proj_match_point_index_set)
  [proj_x_set] -> location transformer/5(proj_x_set)
  [frenet_path_y] -> location transformer/4(frenet_path_y)
  [frenet_path_x] -> location transformer/3(frenet_path_x)
  [y_set] -> location transformer/2(y_set)
  [x_set] -> location transformer/1(x_set)
  index2s/1 -> [index2s]
  proj_kappa_set/1 -> [proj_kappa_set]
  proj_heading_set/1 -> [proj_heading_set]
  proj_y_set/1 -> [proj_y_set]
  proj_x_set/1 -> [proj_x_set]
  proj_match_point_index_set/1 -> [proj_match_point_index_set]
  frenet_path_y/1 -> [frenet_path_y]
  frenet_path_x/1 -> [frenet_path_x]
  ay_set/1 -> [ay_set]
  ax_set/1 -> [ax_set]
  vy_set/1 -> [vy_set]
  vx_set/1 -> [vx_set]
  y_set/1 -> [y_set]
  x_set/1 -> [x_set]

== system planner_contral/decision_planning/EMplanner/obs/Cartesian2Frenet_static ==
  x_set : Inport
  y_set : Inport  Port=2
  vx_set : Inport  Port=3
  vy_set : Inport  Port=4
  ax_set : Inport  Port=5
  ay_set : Inport  Port=6
  frenet_path_x : Inport  Port=7
  frenet_path_y : Inport  Port=8
  proj_match_point_index_set : Inport  Port=9
  proj_x_set : Inport  Port=10
  proj_y_set : Inport  Port=11
  proj_heading_set : Inport  Port=12
  proj_kappa_set : Inport  Port=13
  index2s : Inport  Port=14
  Bus Creator : BusCreator  Inputs=8
  From10 : From  Commented=on  GotoTag=vx_set
  From11 : From  Commented=on  GotoTag=vy_set
  From12 : From  Commented=on  GotoTag=proj_heading_set
  From13 : From  Commented=on  GotoTag=proj_kappa_set
  From14 : From  Commented=on  GotoTag=ax_set
  From15 : From  Commented=on  GotoTag=ay_set
  From16 : From  Commented=on  GotoTag=proj_heading_set
  From17 : From  Commented=on  GotoTag=proj_kappa_set
  From18 : From  Commented=on  GotoTag=l_set
  From19 : From  Commented=on  GotoTag=s_dot_set
  From20 : From  Commented=on  GotoTag=dl_set
  From7 : From  Commented=on  GotoTag=l_set
  MATLAB Function : MATLAB Function  TreatAsAtomicUnit=on
  MATLAB Function1 : MATLAB Function  Commented=on  TreatAsAtomicUnit=on
  MATLAB Function2 : MATLAB Function  Commented=on  TreatAsAtomicUnit=on
  Cartesian2FrenetOut : Outport
  wires:
  Bus Creator/1 -> Cartesian2FrenetOut/1
  [ddl_set] -> Bus Creator/8  "ddl_set"
  [l_dot2_set] -> Bus Creator/7  "l_dot2_set"
  [s_dot2_set] -> Bus Creator/6  "s_dot2_set"
  [dl_set] -> Bus Creator/5  "dl_set"
  [l_dot_set] -> Bus Creator/4  "l_dot_set"
  [s_dot_set] -> Bus Creator/3  "s_dot_set"
  [l_set] -> Bus Creator/2  "l_set"
  [s_set] -> Bus Creator/1  "s_set"
  MATLAB Function2/3(ddl_set) -> [ddl_set]
  MATLAB Function2/2(l_dot2_set) -> [l_dot2_set]
  MATLAB Function2/1(s_dot2_set) -> [s_dot2_set]
  From20/1 -> MATLAB Function2/7(dl_set)
  From19/1 -> MATLAB Function2/6(s_dot_set)
  MATLAB Function1/3(dl_set) -> [dl_set]
  MATLAB Function1/2(l_dot_set) -> [l_dot_set]
  MATLAB Function1/1(s_dot_set) -> [s_dot_set]
  From18/1 -> MATLAB Function2/5(l_set)
  From17/1 -> MATLAB Function2/4(proj_kappa_set)
  From16/1 -> MATLAB Function2/3(proj_heading_set)
  From15/1 -> MATLAB Function2/2(ay_set)
  From14/1 -> MATLAB Function2/1(ax_set)
  From13/1 -> MATLAB Function1/5(proj_kappa_set)
  From12/1 -> MATLAB Function1/4(proj_heading_set)
  From11/1 -> MATLAB Function1/3(vy_set)
  From10/1 -> MATLAB Function1/2(vx_set)
  From7/1 -> MATLAB Function1/1(l_set)
  MATLAB Function/2(l_set) -> [l_set]
  MATLAB Function/1(s_set) -> [s_set]
  [index2s] -> MATLAB Function/9(index2s)
  [proj_heading_set] -> MATLAB Function/7(proj_heading_set)
  [proj_y_set] -> MATLAB Function/6(proj_y_set)
  [proj_match_point_index_set] -> MATLAB Function/8(proj_match_point_index_set)
  [proj_x_set] -> MATLAB Function/5(proj_x_set)
  [frenet_path_y] -> MATLAB Function/4(frenet_path_y)
  [frenet_path_x] -> MATLAB Function/3(frenet_path_x)
  [y_set] -> MATLAB Function/2(y_set)
  [x_set] -> MATLAB Function/1(x_set)
  index2s/1 -> [index2s]
  proj_kappa_set/1 -> [proj_kappa_set]
  proj_heading_set/1 -> [proj_heading_set]
  proj_y_set/1 -> [proj_y_set]
  proj_x_set/1 -> [proj_x_set]
  proj_match_point_index_set/1 -> [proj_match_point_index_set]
  frenet_path_y/1 -> [frenet_path_y]
  frenet_path_x/1 -> [frenet_path_x]
  ay_set/1 -> [ay_set]
  ax_set/1 -> [ax_set]
  vy_set/1 -> [vy_set]
  vx_set/1 -> [vx_set]
  y_set/1 -> [y_set]
  x_set/1 -> [x_set]

== matlab function planner_contral/decision_planning/EMplanner/path planning task/MATLAB Function ==
  data: qp_path_s input; qp_path_s_final output; qp_path_l input; qp_path_dl input; qp_path_ddl input; qp_path_l_final output; qp_path_dl_final output; qp_path_ddl_final output
function [qp_path_s_final,qp_path_l_final, qp_path_dl_final,qp_path_ddl_final] = fcn(qp_path_s,qp_path_l,qp_path_dl,qp_path_ddl)
% 该函数将增密qp_path
n_init = 20;
% 增密的点的个数
n = 501;
% 输出初始化
qp_path_s_final = zeros(n,1);
qp_path_l_final = zeros(n,1);
qp_path_dl_final = zeros(n,1);
qp_path_ddl_final = zeros(n,1);
ds = (qp_path_s(end) - qp_path_s(1))/(n-1);
index = 1;
for i = 1:n
    x = qp_path_s(1) + (i-1) * ds;
    qp_path_s_final(i) = x;
    while x >= qp_path_s(index)
        index = index + 1;
        if index == n_init
            break;
        end
    end
    % while 循环退出的条件是x<qp_path_s(index)，所以x对应的前一个s的编号是index-1 后一个编号是index
    pre = index - 1;
    cur = index;
    % 计算前一个点的l l' l'' ds 和后一个点的 l''
    delta_s = x - qp_path_s(pre);
    l_pre = qp_path_l(pre);
    dl_pre = qp_path_dl(pre);
    ddl_pre = qp_path_ddl(pre);
    ddl_cur = qp_path_ddl(cur);
    % 分段加加速度优化 
    qp_path_l_final(i) = l_pre + dl_pre * delta_s + (1/3)* ddl_pre * delta_s^2 + (1/6) * ddl_cur * delta_s^2;
    qp_path_dl_final(i) = dl_pre + 0.5 * ddl_pre * delta_s + 0.5 * ddl_cur * delta_s;
    qp_path_ddl_final(i) = ddl_pre + (ddl_cur - ddl_pre) * delta_s/(qp_path_s(cur) - qp_path_s(pre));
    %  因为此时x的后一个编号是index 必有x < qp_path_s(index),在下一个循环中x = x + ds 也未必大于
    %  qp_path_s(index)，这样就进入不了while循环，所以index 要回退一位
    index = index - 1;   
end
